simulink model "scheme2"  (R2024a)
settings: Solver=VariableStepAuto  StartTime=0.0  StopTime=30  RelTol=1e-6
values from neighbouring files (symbols this model uses):
  a0 = -2    [main.m]
  a1 = -1    [main.m]
  a2 = 1    [main.m]
  dy0 = 3    [main.m]
  k0 = -3    [main.m]
  k1 = -3    [main.m]
  T = 0.001    [main.m]
  y0 = 2    [main.m]
settings Model: Creator=alexivanov  LastModifiedBy=alexivanov

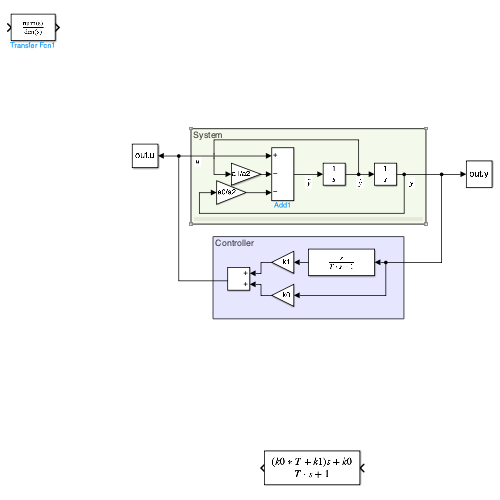
[thumbnail: Simulink's stored preview of the top-level diagram]
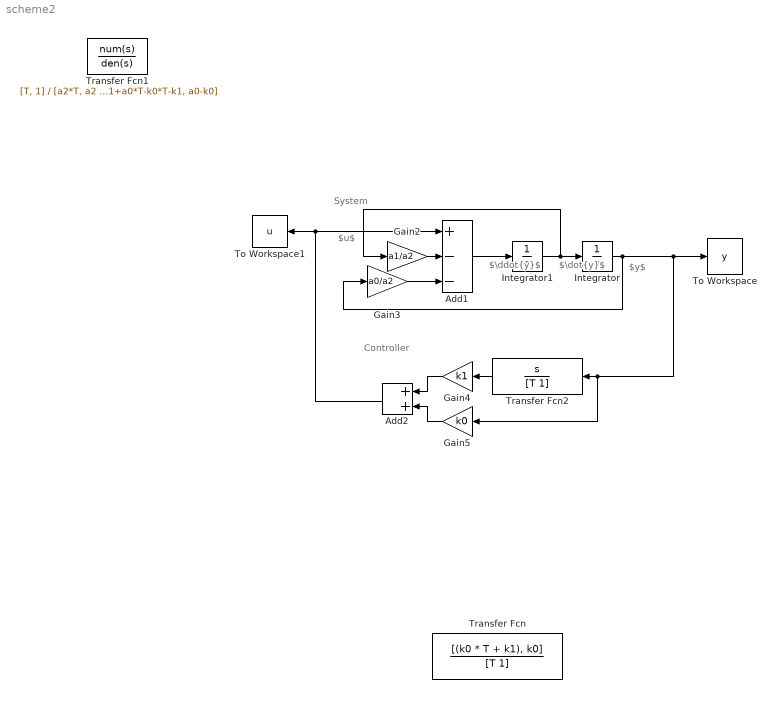
== system scheme2 ==
  note: System
  note: $y$
  note: $\dot{y}$
  note: $\ddot{y}$
  note: $u$
  note: Controller
  Add1 : Sum  Inputs=+--
  Add2 : Sum
  Gain2 : Gain  Gain=a1/a2
  Gain3 : Gain  Gain=a0/a2
  Gain4 : Gain  Gain=k1
  Gain5 : Gain  Gain=k0
  Integrator : Integrator  InitialCondition=y0
  Integrator1 : Integrator  InitialCondition=dy0
  To Workspace : ToWorkspace  VariableName=y  SaveFormat=Timeseries  SampleTime=-1
  To Workspace1 : ToWorkspace  VariableName=u  SaveFormat=Timeseries  SampleTime=-1
  Transfer Fcn : TransferFcn  Numerator=[(k0 * T + k1), k0]  Denominator=[T 1]
  Transfer Fcn1 : TransferFcn  Numerator=[T, 1]  Denominator=[a2*T, a2 + a1*T, a1+a0*T-k0*T-k1, a0-k0]
  Transfer Fcn2 : TransferFcn  Numerator=[1 0]  Denominator=[T 1]
  wires:
  Integrator1/1 -> Gain2/1, Integrator/1
  Add1/1 -> Integrator1/1
  Gain2/1 -> Add1/2
  Gain3/1 -> Add1/3
  Gain4/1 -> Add2/1
  Gain5/1 -> Add2/2
  Transfer Fcn2/1 -> Gain4/1
  Integrator/1 -> Gain5/1, Transfer Fcn2/1, To Workspace/1, Gain3/1
  Add2/1 -> To Workspace1/1, Add1/1
